simulink model "FixedWing_Dynamic_Model_SIL_simulink"  (R2023a)
settings: Solver=ode4  StartTime=0.0  StopTime=timestop  FixedStep=0.004  RelTol=1e-3
model workspace (MAT data in the model file):
  sample_time = 0.004
values from neighbouring files (symbols this model uses):
  env = struct    [InitEnvironment.m]    (also in resultados_autotuning_H200.mat = )
  F_lat = 1    [autotuning.m]    (also in resultados_autotuning_H200.mat)
  F_lon = 1    [autotuning.m]    (also in resultados_autotuning_H200.mat)
  frecuency = 0.012    [PX4_var_controllers.m]    (also in resultados_autotuning_H200.mat)
  g = 9.81    [PX4_var_controllers.m]    (also in resultados_autotuning_H200.mat)
  LC =     [resultados_autotuning_H200.mat]
  mission = [wp]    [PX4_var_controllers.m]    (also in resultados_autotuning_H200.mat = )
  nav = 0    [autotuning.m]    (also in resultados_autotuning_H200.mat)
  nwap = 9    [PX4_var_controllers.m]    (also in resultados_autotuning_H200.mat)
  pitch_D = p(8)    [Error_Medio_Cuadratico_tot.m]    (also in autotuning.m = gaDat3.xmin(8); resultados_autotuning_H200.mat = 0.0563748318956)
  pitch_ff = p(10)    [Error_Medio_Cuadratico_tot.m]    (also in autotuning.m = gaDat3.xmin(10); resultados_autotuning_H200.mat = 0.191071934851)
  pitch_I = p(7)    [Error_Medio_Cuadratico_tot.m]    (also in autotuning.m = gaDat3.xmin(7); resultados_autotuning_H200.mat = 5.51002123548)
  pitch_P = p(6)    [Error_Medio_Cuadratico_tot.m]    (also in autotuning.m = gaDat3.xmin(6); resultados_autotuning_H200.mat = 0.842081867818)
  poswp = [poswp1;poswp2;poswp3;poswp4;poswp5;poswp6;poswp7;poswp8;poswp9]    [PX4_var_controllers.m]    (also in resultados_autotuning_H200.mat = [0 203.689232032 39.9384744604 259.790159417 479.641844374 3)
  ref_height = 171    [resultados_autotuning_H200.mat]
  ref_lat = 39.4973880749    [resultados_autotuning_H200.mat]
  ref_lon = -0.626812248872    [resultados_autotuning_H200.mat]
  roll_D = p(3)    [Error_Medio_Cuadratico_lat.m]    (also in Error_Medio_Cuadratico_tot.m; autotuning.m = gaDat3.xmin(3); resultados_autotuning_H200.mat = 0.0337053005157)
  roll_ff = p(5)    [Error_Medio_Cuadratico_lat.m]    (also in Error_Medio_Cuadratico_tot.m; autotuning.m = gaDat3.xmin(5); resultados_autotuning_H200.mat = 0.350805641616)
  roll_I = p(2)    [Error_Medio_Cuadratico_lat.m]    (also in Error_Medio_Cuadratico_tot.m; autotuning.m = gaDat3.xmin(2); resultados_autotuning_H200.mat = 5.74910821603)
  roll_P = p(1)    [Error_Medio_Cuadratico_lat.m]    (also in Error_Medio_Cuadratico_tot.m; autotuning.m = gaDat3.xmin(1); resultados_autotuning_H200.mat = 0.613573974385)
  tc_pitch = p(9)    [Error_Medio_Cuadratico_tot.m]    (also in autotuning.m = gaDat3.xmin(9); resultados_autotuning_H200.mat = 0.651709962584)
  tc_roll = p(4)    [Error_Medio_Cuadratico_lat.m]    (also in Error_Medio_Cuadratico_tot.m; autotuning.m = gaDat3.xmin(4); resultados_autotuning_H200.mat = 0.630975334126)
  TEBCL =     [resultados_autotuning_H200.mat]
  TECL =     [resultados_autotuning_H200.mat]
  TECS =     [resultados_autotuning_H200.mat]
  throttle_sp = 0.6    [autotuning.m]    (also in resultados_autotuning_H200.mat)
  uavData = struct    [InitFixedWingParam.m]    (also in resultados_autotuning_H200.mat = )
  V_cruise = [15,15,15,20,25,25,20,15,15]    [PX4_var_controllers.m]    (also in resultados_autotuning_H200.mat = [15 15 15 20 25 25 20 15 15])
  yaw_D = p(8)    [Error_Medio_Cuadratico_lat.m]    (also in Error_Medio_Cuadratico_tot.m = p(13); autotuning.m = gaDat3.xmin(13); resultados_autotuning_H200.mat = 0.366142516918)
  yaw_ff = p(9)    [Error_Medio_Cuadratico_lat.m]    (also in Error_Medio_Cuadratico_tot.m = p(14); autotuning.m = gaDat3.xmin(14); resultados_autotuning_H200.mat = 1.32395168)
  yaw_I = p(7)    [Error_Medio_Cuadratico_lat.m]    (also in Error_Medio_Cuadratico_tot.m = p(12); autotuning.m = gaDat3.xmin(12); resultados_autotuning_H200.mat = 9.97252106698)
  yaw_P = p(6)    [Error_Medio_Cuadratico_lat.m]    (also in Error_Medio_Cuadratico_tot.m = p(11); autotuning.m = gaDat3.xmin(11); resultados_autotuning_H200.mat = 9.79447138521)
undefined symbols (not defined in the file or in its folder): DiscIntNeverNeededParam, Earth, WGS84
libraries: aerolibactuator x5, aerolibasang x4, slpidlib x3, uavalgslib x2, aerolibatmos2 x2, shared6dof x1, aerolibtransform2 x1, simulink_extras x1
(part 1 of 3)
settings Model: Creator=kboychev  LastModifiedBy=user
settings OptimizationCC: ReuseModelBlockBuffer=off  ZeroExternalMemoryAtStartup=off  ZeroInternalMemoryAtStartup=off
settings ModelReferenceCC: EnableRefExpFcnMdlSchedulingChecks=on
settings RTWCC: Toolchain=Microsoft Visual C++ 2017 v15.0 | nmake (64-bit Windows)  TargetLang=C++
settings GRTTargetCC: TargetLangStandard=C++11 (ISO)  CodeInterfacePackaging=C++ class

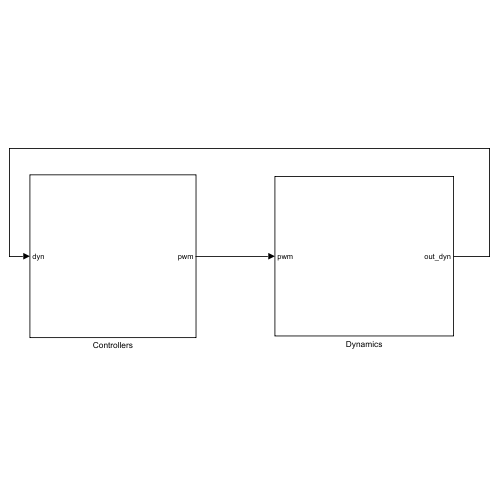
[thumbnail: Simulink's stored preview of the top-level diagram]
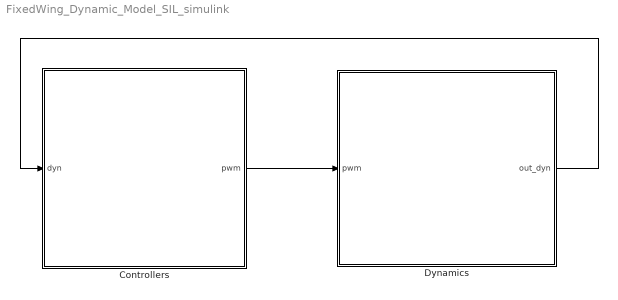
== system FixedWing_Dynamic_Model_SIL_simulink ==
  Controllers : Subsystem
  Dynamics : Subsystem
  wires:
  Dynamics/1(out_dyn) -> Controllers/1(dyn)
  Controllers/1(pwm) -> Dynamics/1(pwm)

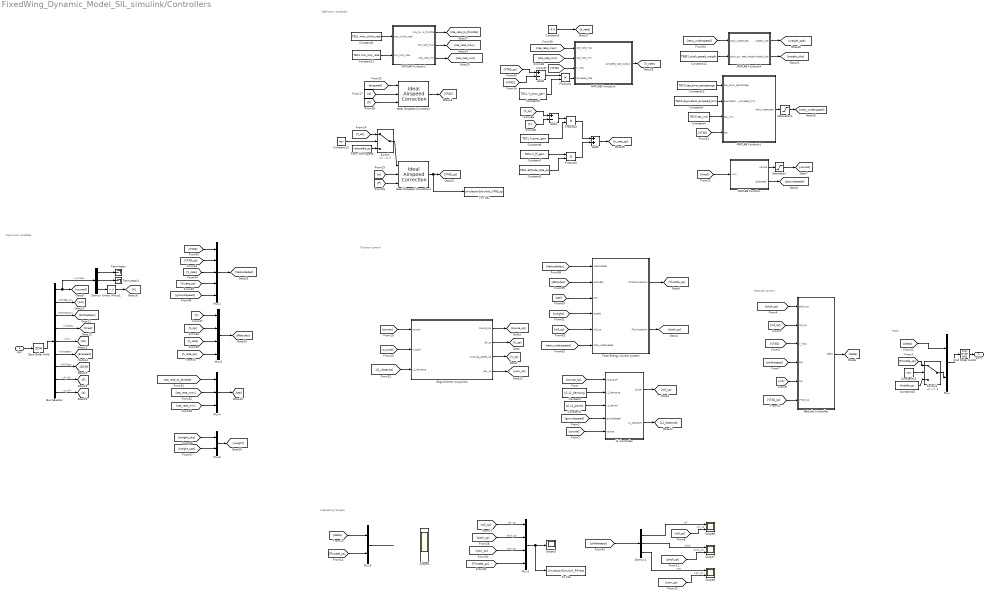
== system FixedWing_Dynamic_Model_SIL_simulink/Controllers ==
  note: Interesting Scopes
  note: Definition Variables
  note: Input and variables
  note: PWM
  note: Attitude control
  note: Position control
  dyn : Inport
  Add3 : Sum  Inputs=+-
  Add4 : Sum  Inputs=+-
  Add5 : Sum
  Attitude Controller : Subsystem
  Bus Selector : BusSelector  OutputSignals=xyzned,omega_b,phithetapsi,Vbned,Vb,airspeed,DCMbe,P_inf,a_inf
  Constant : Constant  Value=LC.L1_damping  SampleTime=frecuency
  Constant1 : Constant  Value=LC.L1_period  SampleTime=frecuency
  Constant10 : Constant  Value=TECS.tas_error_percetange  SampleTime=frecuency
  Constant11 : Constant  Value=TECL.min_sink_rate  SampleTime=frecuency
  Constant12 : Constant  Value=TEBCL.pitch_speed_weight  SampleTime=frecuency
  Constant13 : Constant  Value=nav  SampleTime=frecuency
  Constant15 : Constant  Value=nav  SampleTime=frecuency
  Constant16 : Constant  Value=throttle_sp  SampleTime=frecuency
  Constant2 : Constant  Value=TECL.altitude_rate_sp  SampleTime=frecuency
  Constant3 : Constant  Value=-0.5  SampleTime=frecuency
  Constant4 : Constant  Value=TECS.tas_min  SampleTime=frecuency
  Constant5 : Constant  Value=TECL.V_error_gain  SampleTime=frecuency
  Constant6 : Constant  Value=TECL.h_error_gain  SampleTime=frecuency
  Constant7 : Constant  Value=TECL.h_ff_gain  SampleTime=frecuency
  Constant8 : Constant  Value=TECL.max_climb_rate  SampleTime=frecuency
  Constant9 : Constant  Value=TECS.equivalent_airspeed_trim  SampleTime=frecuency
  Demux : Demux  Outputs=3
  Demux1 : Demux  Outputs=3
  First Order Hold1 : FirstOrderHold  ErrorTolerance=inf  AllowContinuousInput=on
  From Workspace : FromWorkspace  VariableName=velocidad_sp  SampleTime=frecuency
  Ideal Airspeed Correction : aerolibasang/Ideal Airspeed Correction  units=Metric (MKS)  vel_in=EAS  vel_out_tas=EAS  vel_out_eas=TAS  vel_out_cas=TAS  method=Table Lookup  SubOnly=off  action=None
  Ideal Airspeed Correction1 : aerolibasang/Ideal Airspeed Correction  units=Metric (MKS)  vel_in=EAS  vel_out_tas=EAS  vel_out_eas=TAS  vel_out_cas=TAS  method=Table Lookup  SubOnly=off  action=None
  L1 Controller : Subsystem
  MATLAB Function : MATLAB Function  TreatAsAtomicUnit=on  SystemSampleTime=frecuency
  MATLAB Function1 : MATLAB Function  TreatAsAtomicUnit=on  SystemSampleTime=frecuency
  MATLAB Function2 : MATLAB Function  TreatAsAtomicUnit=on  SystemSampleTime=frecuency
  MATLAB Function3 : MATLAB Function  TreatAsAtomicUnit=on  SystemSampleTime=frecuency
  MATLAB Function4 : MATLAB Function  TreatAsAtomicUnit=on  SystemSampleTime=frecuency
  Mux : Mux  Inputs=2
  Mux1 : Mux
  Mux2 : Mux  Inputs=5
  Mux3 : Mux
  Mux4 : Mux  Inputs=3
  Mux5 : Mux  Inputs=2
  Mux6 : Mux  Inputs=2
  Product2 : Product
  Product3 : Product
  Product4 : Product
  Saturation : Saturate  UpperLimit=pi  LowerLimit=-pi
  Saturation1 : Saturate  UpperLimit=1  LowerLimit=0
  Scope3 : Scope
  Scope4 : Scope  NumInputPorts=4
  Scope6 : Scope  NumInputPorts=2
  Scope7 : Scope  NumInputPorts=2
  Scope8 : Scope  NumInputPorts=2
  Seguimiento waypoints : Subsystem
  Switch : Switch  Criteria=u2 ~= 0  SaturateOnIntegerOverflow=off  InputSameDT=off
  Switch1 : Switch  Criteria=u2 ~= 0  SaturateOnIntegerOverflow=off  InputSameDT=off
  Terminator : Terminator
  Terminator1 : Terminator
  To File : ToFile  Filename=simulacionSimulink_RPYest  SaveFormat=Timeseries
  To File1 : ToFile  Filename=simulacionSimulink_VTAS_sp  SaveFormat=Timeseries
  Total Energy control system : Subsystem
  Unary Minus1 : UnaryMinus
  Zero-Order Hold : ZeroOrderHold  SampleTime=frecuency
  pwm : Outport
  wires:
  Seguimiento waypoints/2(alt_sp) -> [h_sp]
  Seguimiento waypoints/3(cruising_speed_sp) -> [V_sp]
  Seguimiento waypoints/1(Course_sp) -> [course_sp]
  [course] -> L1 Controller/5(course)
  Total Energy control system/1(Throttle setpoint) -> [Throttle_sp]
  Total Energy control system/2(Pitch setpoint) -> [pitch_sp]
  [pitch_sp] -> Attitude Controller/1(pitch_sp)
  [roll_sp] -> Attitude Controller/2(roll_sp)
  [VTAS] -> Attitude Controller/3(V_TAS)
  [phithetapsi] -> Attitude Controller/4("RPY ")
  [wb] -> Attitude Controller/5(wb)
  [VTAS_sp] -> Attitude Controller/6(VTAS_sp)
  Attitude Controller/1(delta) -> [delta]
  [course] -> Seguimiento waypoints/1(course)
  [xyzned] -> Seguimiento waypoints/2(xyzgnd)
  MATLAB Function/1(course) -> Saturation/1
  Bus Selector/1 -> Demux/1, [xyzned]  "<xyzned>"
  Bus Selector/2 -> [wb]  "<omega_b>"
  Bus Selector/3 -> [phithetapsi]  "<phithetapsi>"
  Bus Selector/4 -> [Vned]  "<Vbned>"
  Bus Selector/5 -> [Vb]  "<Vb>"
  Bus Selector/6 -> [airspeed]  "<airspeed>"
  Bus Selector/7 -> [DCM]  "<DCMbe>"
  Bus Selector/8 -> [P]  "<P_inf>"
  Bus Selector/9 -> [a]  "<a_inf>"
  [a] -> Ideal Airspeed Correction/2
  [P] -> Ideal Airspeed Correction/3
  [airspeed] -> Ideal Airspeed Correction/1
  [P] -> Ideal Airspeed Correction1/3
  [a] -> Ideal Airspeed Correction1/2
  Ideal Airspeed Correction1/1 -> To File1/1, [VTAS_sp]
  Demux/1 -> Terminator/1
  Demux/2 -> Terminator1/1
  Demux/3 -> Unary Minus1/1
  Unary Minus1/1 -> [h]
  L1 Controller/2(L1_distance) -> [L1_distance]
  L1 Controller/1(roll SP) -> [roll_sp]
  [groundspeed] -> L1 Controller/4(groundSpeed)
  MATLAB Function/2(gndspeed) -> [groundspeed]
  Seguimiento waypoints/4(yaw_sp) -> [yaw_sp]
  [roll_sp] -> Mux1/1  "roll_sp"
  [pitch_sp] -> Mux1/2  "pitch_sp"
  [yaw_sp] -> Mux1/3  "yaw_sp"
  [Throttle_sp] -> Mux1/4
  Ideal Airspeed Correction/1 -> [VTAS]
  Mux1/1 -> Scope3/1, To File/1
  Saturation/1 -> [course]
  [Vned] -> MATLAB Function/1(vxyz)
  Demux1/2 -> Scope7/1  "pitch"
  Demux1/3 -> Scope8/1  "yaw"
  dyn/1 -> Zero-Order Hold/1
  Mux/1 -> First Order Hold1/1
  Zero-Order Hold/1 -> Bus Selector/1
  Constant/1 -> L1 Controller/2(L1_damping)
  Constant1/1 -> L1 Controller/3(L1_period)
  Demux1/1 -> Scope6/1  "roll"
  First Order Hold1/1 -> pwm/1
  [delta] -> Mux/1
  [course_sp] -> L1 Controller/1(course SP)
  [L1_distance] -> Seguimiento waypoints/3(L1_distance)
  Saturation1/1 -> [ratio_underspeed]
  Constant9/1 -> MATLAB Function1/2(equivalent_airspeed_trim)
  Constant8/1 -> MATLAB Function2/1(max_climb_rate)
  Constant4/1 -> MATLAB Function1/3(tas_min)
  Constant10/1 -> MATLAB Function1/1(tas_error_percentage)
  MATLAB Function1/1(ratio_undersped) -> Saturation1/1
  Constant11/1 -> MATLAB Function2/2(min_sink_rate)
  [VTAS] -> MATLAB Function1/4(tas)
  MATLAB Function2/2(ste_rate_max) -> [ste_rate_max]
  MATLAB Function2/3(ste_rate_min) -> [ste_rate_min]
  MATLAB Function2/1(ste_rate_to_throttle) -> [ste_rate_to_throttle]
  [VTAS] -> MATLAB Function3/3(V_TAS)
  [ste_rate_max] -> MATLAB Function3/1(ste_rate_max)
  [h] -> Add4/2
  [ste_rate_min] -> MATLAB Function3/2(ste_rate_min)
  Constant5/1 -> Product2/2
  Constant6/1 -> Product3/2
  Product4/1 -> Add5/2
  [h_sp] -> Add4/1
  Add3/1 -> Product2/1
  Product2/1 -> MATLAB Function3/4(airspeed_rate)
  [VTAS] -> Add3/2
  Product3/1 -> Add5/1
  Constant7/1 -> Product4/1
  [VTAS_sp] -> Add3/1
  Constant2/1 -> Product4/2
  Add4/1 -> Product3/1
  MATLAB Function3/1(airspeed_rate_output) -> [V_rate]
  [ratio_underspeed] -> MATLAB Function4/1(ratio_undersped)
  Constant12/1 -> MATLAB Function4/2(pitch_speed_weight)
  MATLAB Function4/1(weight_spe) -> [weight_spe]
  MATLAB Function4/2(weight_ske) -> [weight_ske]
  [phithetapsi] -> Demux1/1
  Mux2/1 -> [Velocidades]
  [VTAS] -> Mux2/1
  [VTAS_sp] -> Mux2/2
  [V_rate] -> Mux2/3
  [V_rate_sp] -> Mux2/4
  [groundspeed] -> Mux2/5
  Mux3/1 -> [Altitudes]
  [h] -> Mux3/1
  [h_sp] -> Mux3/2
  [h_rate] -> Mux3/3
  [h_rate_sp] -> Mux3/4
  Mux4/1 -> [ste]
  [ste_rate_to_throttle] -> Mux4/1
  [ste_rate_max] -> Mux4/2
  [ste_rate_min] -> Mux4/3
  Mux6/1 -> [weight]
  [weight_spe] -> Mux6/2
  [weight_ske] -> Mux6/1
  [Velocidades] -> Total Energy control system/1(Velocidades)
  [Altitudes] -> Total Energy control system/2(Altitudes)
  [ste] -> Total Energy control system/3(ste)
  [weight] -> Total Energy control system/4(weight)
  [roll_sp] -> Total Energy control system/5(roll_sp)
  [ratio_underspeed] -> Total Energy control system/6(ratio_underspeed)
  Add5/1 -> [h_rate_sp]
  Constant3/1 -> [h_rate]
  [roll_sp] -> Scope6/2  "roll_sp"
  [pitch_sp] -> Scope7/2  "pitch_sp"
  [yaw_sp] -> Scope8/2  "yaw_sp"
  Mux5/1 -> ?
  [delta] -> Mux5/1
  [Throttle_sp] -> Mux5/2
  ? -> Scope4/3  "dR"
  ? -> Scope4/1  "dE"
  ? -> Scope4/2  "dA"
  ? -> Scope4/4  "dT"
  [V_sp] -> Switch/1
  Switch/1 -> Ideal Airspeed Correction1/1
  Constant13/1 -> Switch/2
  From Workspace/1 -> Switch/3
  Constant16/1 -> Switch1/3
  Constant15/1 -> Switch1/2
  [Throttle_sp] -> Switch1/1
  Switch1/1 -> Mux/2

== system FixedWing_Dynamic_Model_SIL_simulink/Dynamics ==
  note: Pixhawk SIL Connector for Simulink
      | Fixed-Wing Dynamics
  pwm : Inport
  Bus Selector : BusSelector  OutputSignals=mulh,phithetapsi,Vbned,xyzned,Vb,omega_b,g,B
  Demux : Demux  Outputs=3
  Display{,1..5,10..11,13} (9 alike) : Display
  H200 Fixed-wing UAV Dynamics : Subsystem
  Radians to Degrees2 : simulink_extras/Transformations/Radians to Degrees
  Scope2 : Scope
  Unary Minus : UnaryMinus
  XY Graph : Record  FileSettingsInternal="{\"entries\":[{\"content\":{\"excelSettings\":{\"content\":{},\"type\":\"Streamout.ExcelSettings\"}},\"type\":\"Streamout.FileSettingStorage\",\"uuid\":\"\"}],\"packageUris\":[\"http:\\/\\/schema.mathworks.com\\/mf0\\/streamout_blocks\\/R2020a\"],\"version\":\"1.0\"}"  Layout=[1 1]  SignalsInternal="{\"entries\":[{\"content\":{\"signals\":[{\"content\":{\"blockPath\":[],\"dimensions\":[1],\"domain\":\"\",\"lineColor\":\"#a2142f\",\"plots\":[1],\"port\":1,\"signalID\":86,\"signalName\":\"Demux:2\"},\"type\":\"RecordBlkView.Signal\",\"uuid\":\"\"},{\"content\":{\"blockPath\":[],\"dimensions\":[1],\"domain\":\"\",\"lineColor\":\"#139fff\",\"plots\":[1],\"port\":2,\"signalID\":89,\"signalName\":\"Demux:1\"},\"type\":\"RecordBlkView.Signal\",\"uuid\":\"\"}]},\"type\":\"RecordBlkView.InputSignals\",\"uuid\":\"\"}],\"packageUris\":[\"http:\\/\\/schema.mathworks.com\\/mf0\\/streamout_blocks\\/R2020a\"],\"version\":\"1.0\"}"  VisualizationBindings="{\"xyplotplugin\":{\"info\":[{\"series\":[{\"bindingParametersList\":[{\"parameter\":\"X-Axis\",\"signalID\":86,\"signalName\":\"Demux:2\"},{\"parameter\":\"Y-Axis\",\"signalID\":89,\"signalName\":\"Demux:1\"}],\"seriesID\":12918}],\"subplotID\":1}]}}"  CompatibilityTag=XY
  XY Graph1 : Record  FileSettingsInternal="{\"entries\":[{\"content\":{\"excelSettings\":{\"content\":{},\"type\":\"Streamout.ExcelSettings\"}},\"type\":\"Streamout.FileSettingStorage\",\"uuid\":\"\"}],\"packageUris\":[\"http:\\/\\/schema.mathworks.com\\/mf0\\/streamout_blocks\\/R2020a\"],\"version\":\"1.0\"}"  Layout=[1 1]  SignalsInternal="{\"entries\":[{\"content\":{\"signals\":[{\"content\":{\"blockPath\":[],\"dimensions\":[1],\"domain\":\"\",\"lineColor\":\"#a2142f\",\"plots\":[1],\"port\":1,\"signalID\":78,\"signalName\":\"Demux:1\"},\"type\":\"RecordBlkView.Signal\",\"uuid\":\"\"},{\"content\":{\"blockPath\":[],\"dimensions\":[1],\"domain\":\"\",\"lineColor\":\"#139fff\",\"plots\":[1],\"port\":2,\"signalID\":81,\"signalName\":\"Unary Minus\"},\"type\":\"RecordBlkView.Signal\",\"uuid\":\"\"}]},\"type\":\"RecordBlkView.InputSignals\",\"uuid\":\"\"}],\"packageUris\":[\"http:\\/\\/schema.mathworks.com\\/mf0\\/streamout_blocks\\/R2020a\"],\"version\":\"1.0\"}"  VisualizationBindings="{\"xyplotplugin\":{\"info\":[{\"series\":[{\"bindingParametersList\":[{\"parameter\":\"X-Axis\",\"signalID\":78,\"signalName\":\"Demux:1\"},{\"parameter\":\"Y-Axis\",\"signalID\":81,\"signalName\":\"Unary Minus\"}],\"seriesID\":30530}],\"subplotID\":1}]}}"  CompatibilityTag=XY
  save to file : Subsystem
  out_dyn : Outport
  wires:
  Bus Selector/4 -> Demux/1, Display10/1  "<xyzned>"
  Radians to Degrees2/1 -> Display1/1, Scope2/1
  Bus Selector/1 -> Display/1  "<mulh>"
  Bus Selector/5 -> Display3/1  "<Vb>"
  Bus Selector/7 -> Display13/1  "<g>"
  Bus Selector/8 -> Display11/1  "<B>"
  Bus Selector/3 -> Display2/1  "<Vbned>"
  Bus Selector/6 -> Display4/1  "<omega_b>"
  Bus Selector/2 -> Radians to Degrees2/1  "<phithetapsi>"
  H200 Fixed-wing UAV Dynamics/1(out) -> out_dyn/1, save to file/2(out), Bus Selector/1
  Demux/1 -> XY Graph/2, XY Graph1/1
  Demux/3 -> Unary Minus/1
  Unary Minus/1 -> XY Graph1/2
  Demux/2 -> XY Graph/1
  pwm/1 -> H200 Fixed-wing UAV Dynamics/1(pwm), Display5/1, save to file/1(pwm)

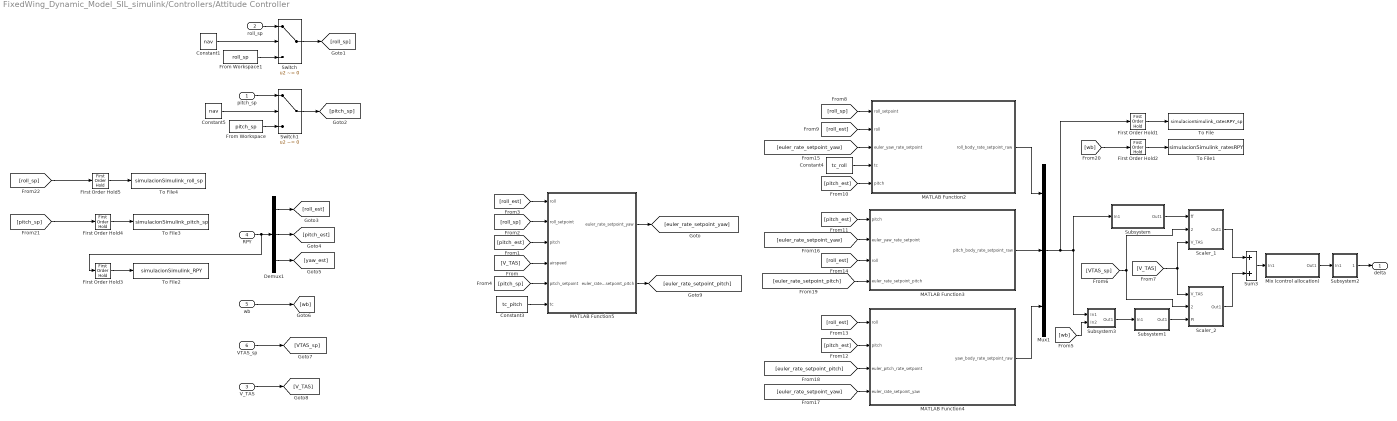
== system FixedWing_Dynamic_Model_SIL_simulink/Controllers/Attitude Controller ==
  pitch_sp : Inport  SampleTime=frecuency
  roll_sp : Inport  Port=2  SampleTime=frecuency
  V_TAS : Inport  Port=3  SampleTime=frecuency
  "RPY " : Inport  Port=4  SampleTime=frecuency
  wb : Inport  Port=5  SampleTime=frecuency
  VTAS_sp : Inport  Port=6  SampleTime=frecuency
  Constant1 : Constant  Value=nav  SampleTime=frecuency
  Constant3 : Constant  Value=tc_pitch  SampleTime=frecuency
  Constant4 : Constant  Value=tc_roll  SampleTime=frecuency
  Constant5 : Constant  Value=nav  SampleTime=frecuency
  Demux1 : Demux  Outputs=3
  First Order Hold{1..5} (5 alike) : FirstOrderHold  ErrorTolerance=inf  AllowContinuousInput=on
  From Workspace : FromWorkspace  VariableName=pitch_sp  SampleTime=frecuency
  From Workspace1 : FromWorkspace  VariableName=roll_sp  SampleTime=frecuency
  MATLAB Function2 : MATLAB Function  TreatAsAtomicUnit=on  SystemSampleTime=frecuency
  MATLAB Function3 : MATLAB Function  TreatAsAtomicUnit=on  SystemSampleTime=frecuency
  MATLAB Function4 : MATLAB Function  TreatAsAtomicUnit=on  SystemSampleTime=frecuency
  MATLAB Function5 : MATLAB Function  TreatAsAtomicUnit=on  SystemSampleTime=frecuency
  Mix (control allocation) : Subsystem
  Mux1 : Mux  Inputs=3
  Scaler_1 : Subsystem
  Scaler_2 : Subsystem
  Subsystem : Subsystem
  Subsystem1 : Subsystem
  Subsystem2 : Subsystem
  Subsystem3 : Subsystem
  Sum3 : Sum
  Switch : Switch  Criteria=u2 ~= 0  SaturateOnIntegerOverflow=off  InputSameDT=off
  Switch1 : Switch  Criteria=u2 ~= 0  SaturateOnIntegerOverflow=off  InputSameDT=off
  To File : ToFile  Filename=simulacionSimulink_ratesRPY_sp  SaveFormat=Timeseries
  To File1 : ToFile  Filename=simulacionSimulink_ratesRPY  SaveFormat=Timeseries
  To File2 : ToFile  Filename=simulacionSimulink_RPY  SaveFormat=Timeseries
  To File3 : ToFile  Filename=simulacionSimulink_pitch_sp  SaveFormat=Timeseries
  To File4 : ToFile  Filename=simulacionSimulink_roll_sp  SaveFormat=Timeseries
  delta : Outport  SampleTime=frecuency
  wires:
  Scaler_1/1(Out1) -> Sum3/1
  Subsystem3/1(Out1) -> Subsystem1/1(In1)
  Subsystem/1(Out1) -> Scaler_1/1(ff)
  Mix (control allocation)/1(Out1) -> Subsystem2/1(In1)
  Sum3/1 -> Mix (control allocation)/1(In1)
  Subsystem2/1(Out1) -> delta/1
  Scaler_2/1(Out1) -> Sum3/2
  Subsystem1/1(Out1) -> Scaler_2/3(PI)
  "RPY "/1 -> First Order Hold3/1, Demux1/1
  Constant3/1 -> MATLAB Function5/6(tc)
  Constant4/1 -> MATLAB Function2/4(tc)
  [V_TAS] -> MATLAB Function5/4(airspeed)
  MATLAB Function2/1(roll_body_rate_setpoint_raw) -> Mux1/1
  MATLAB Function3/1(pitch_body_rate_setpoint_raw) -> Mux1/2
  MATLAB Function4/1(yaw_body_rate_setpoint_raw) -> Mux1/3
  Mux1/1 -> First Order Hold1/1, Subsystem3/1(In1), Subsystem/1(In1)
  First Order Hold1/1 -> To File/1
  Demux1/1 -> [roll_est]
  Demux1/2 -> [pitch_est]
  Demux1/3 -> [yaw_est]
  wb/1 -> [wb]
  VTAS_sp/1 -> [VTAS_sp]
  V_TAS/1 -> [V_TAS]
  [roll_est] -> MATLAB Function5/1(roll)
  [roll_sp] -> MATLAB Function5/2(roll_setpoint)
  [pitch_est] -> MATLAB Function5/3(pitch)
  [pitch_sp] -> MATLAB Function5/5(pitch_setpoint)
  [wb] -> Subsystem3/2(In2)
  [VTAS_sp] -> Scaler_2/2(VTAS_sp), Scaler_1/2(VTAS_sp)
  [V_TAS] -> Scaler_2/1(V_TAS), Scaler_1/3(V_TAS)
  MATLAB Function5/2(euler_rate_setpoint_pitch) -> [euler_rate_setpoint_pitch]
  MATLAB Function5/1(euler_rate_setpoint_yaw) -> [euler_rate_setpoint_yaw]
  [roll_sp] -> MATLAB Function2/1(roll_setpoint)
  [roll_est] -> MATLAB Function2/2(roll)
  [pitch_est] -> MATLAB Function2/5(pitch)
  [pitch_est] -> MATLAB Function3/1(pitch)
  [pitch_est] -> MATLAB Function4/2(pitch)
  [roll_est] -> MATLAB Function4/1(roll)
  [roll_est] -> MATLAB Function3/3(roll)
  [euler_rate_setpoint_yaw] -> MATLAB Function2/3(euler_yaw_rate_setpoint)
  [euler_rate_setpoint_yaw] -> MATLAB Function3/2(euler_yaw_rate_setpoint)
  [euler_rate_setpoint_yaw] -> MATLAB Function4/4(euler_rate_setpoint_yaw)
  [euler_rate_setpoint_pitch] -> MATLAB Function3/4(euler_rate_setpoint_pitch)
  [euler_rate_setpoint_pitch] -> MATLAB Function4/3(euler_pitch_rate_setpoint)
  First Order Hold2/1 -> To File1/1
  [wb] -> First Order Hold2/1
  First Order Hold3/1 -> To File2/1
  First Order Hold4/1 -> To File3/1
  [roll_sp] -> First Order Hold5/1
  First Order Hold5/1 -> To File4/1
  [pitch_sp] -> First Order Hold4/1
  roll_sp/1 -> Switch/1
  Switch/1 -> [roll_sp]
  From Workspace1/1 -> Switch/3
  Constant1/1 -> Switch/2
  Switch1/1 -> [pitch_sp]
  pitch_sp/1 -> Switch1/1
  Constant5/1 -> Switch1/2
  From Workspace/1 -> Switch1/3

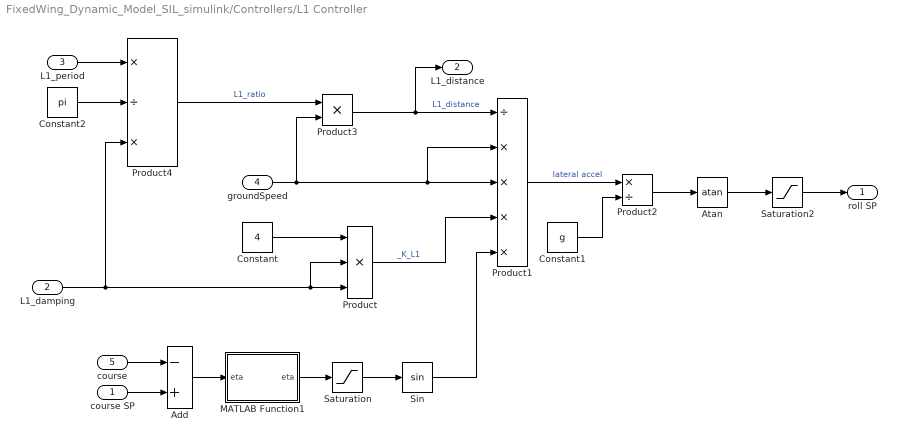
== system FixedWing_Dynamic_Model_SIL_simulink/Controllers/L1 Controller ==
  course SP : Inport  SampleTime=frecuency
  L1_damping : Inport  Port=2  SampleTime=frecuency
  L1_period : Inport  Port=3  SampleTime=frecuency
  groundSpeed : Inport  Port=4  SampleTime=frecuency
  course : Inport  Port=5  SampleTime=frecuency
  Add : Sum  Inputs=-+
  Atan : Trigonometry  Operator=atan
  Constant : Constant  Value=4  SampleTime=frecuency
  Constant1 : Constant  Value=g  SampleTime=frecuency
  Constant2 : Constant  Value=pi  SampleTime=frecuency
  MATLAB Function1 : MATLAB Function  TreatAsAtomicUnit=on  SystemSampleTime=frecuency
  Product : Product  Inputs=3
  Product1 : Product  Inputs=/****
  Product2 : Product  Inputs=*/
  Product3 : Product
  Product4 : Product  Inputs=*/*
  Saturation : Saturate  UpperLimit=pi/2  LowerLimit=-pi/2
  Saturation2 : Saturate  UpperLimit=LC.roll_max  LowerLimit=LC.roll_min
  Sin : Trigonometry
  roll SP : Outport  SampleTime=frecuency
  L1_distance : Outport  Port=2  SampleTime=frecuency
  wires:
  Constant/1 -> Product/1
  L1_damping/1 -> Product4/3, Product/3, Product/2
  groundSpeed/1 -> Product3/2, Product1/2, Product1/3
  Product/1 -> Product1/4  "_K_L1"
  Product1/1 -> Product2/1  "lateral accel"
  Product2/1 -> Atan/1
  Product4/1 -> Product3/1  "L1_ratio"
  L1_period/1 -> Product4/1
  Constant2/1 -> Product4/2
  Constant1/1 -> Product2/2
  Atan/1 -> Saturation2/1
  Sin/1 -> Product1/5
  Product3/1 -> L1_distance/1, Product1/1  "L1_distance"
  Saturation2/1 -> roll SP/1
  Add/1 -> MATLAB Function1/1("eta ")
  MATLAB Function1/1(eta) -> Saturation/1
  Saturation/1 -> Sin/1
  course/1 -> Add/1
  course SP/1 -> Add/2

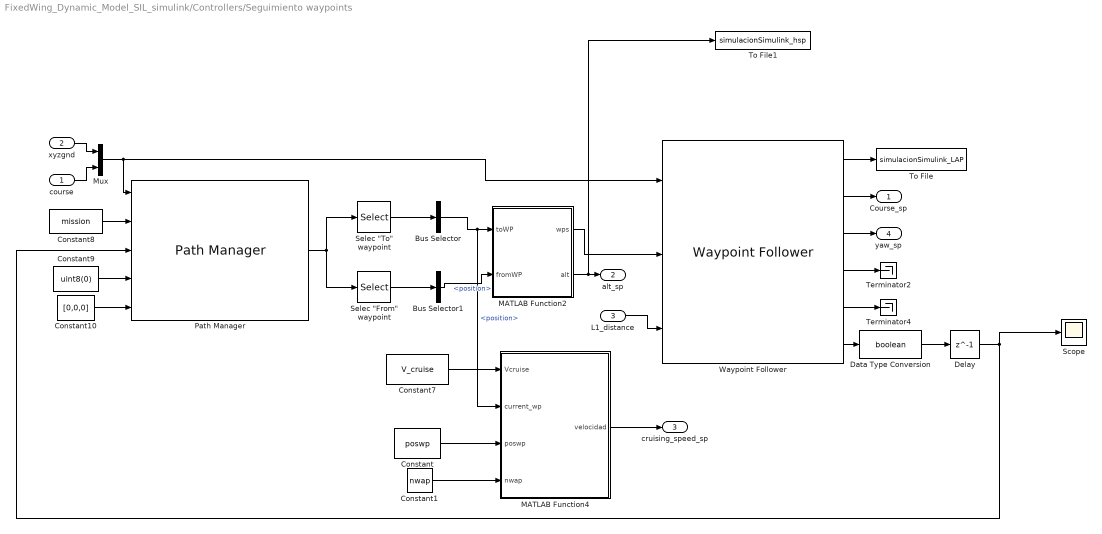
== system FixedWing_Dynamic_Model_SIL_simulink/Controllers/Seguimiento waypoints ==
  course : Inport  SampleTime=frecuency
  xyzgnd : Inport  Port=2  SampleTime=frecuency
  L1_distance : Inport  Port=3  SampleTime=frecuency
  Bus Selector : BusSelector  OutputSignals=position
  Bus Selector1 : BusSelector  OutputSignals=position
  Constant : Constant  Value=poswp  SampleTime=frecuency
  Constant1 : Constant  Value=nwap  SampleTime=frecuency
  Constant10 : Constant  Value=[0,0,0]  SampleTime=frecuency
  Constant7 : Constant  Value=V_cruise  SampleTime=frecuency
  Constant8 : Constant  Value=mission  OutDataTypeStr=Bus: UAVPathManagerBus  SampleTime=frecuency
  Constant9 : Constant  Value=uint8(0)  SampleTime=frecuency
  Data Type Conversion : DataTypeConversion  OutDataTypeStr=boolean  SaturateOnIntegerOverflow=off  RndMeth=Floor
  Delay : Delay  DelayLength=1  SampleTime=frecuency
  MATLAB Function2 : MATLAB Function  TreatAsAtomicUnit=on  SystemSampleTime=frecuency
  MATLAB Function4 : MATLAB Function  TreatAsAtomicUnit=on  SystemSampleTime=frecuency
  Mux : Mux  Inputs=2
  Path Manager : uavalgslib/Path Manager  UAVType=fixed-wing  LoiterRadius=transitionRadius  dataType=double  inputBusName='UAVPathManagerBus'  SimulateUsing=Interpreted execution
  Scope : Scope
  "Selec \"From\" waypoint" : Selector  InputPortWidth=2  IndexOptions=Index vector (dialog)  Indices=2  OutputSizes=1
  "Selec \"To\" waypoint" : Selector  InputPortWidth=2  IndexOptions=Index vector (dialog)  Indices=1  OutputSizes=1
  Terminator2 : Terminator
  Terminator4 : Terminator
  To File : ToFile  Filename=simulacionSimulink_LAP  SaveFormat=Timeseries
  To File1 : ToFile  Filename=simulacionSimulink_hsp  SaveFormat=Timeseries
  Waypoint Follower : uavalgslib/Waypoint Follower  UAVType=fixed-wing  StartFrom=first  TransitionRadiusSource=internal  TransitionRadius=transitionRadius  MinLookaheadDistance=20  YawInput=off  ShowCrossTrackErrorOutput=on  ShowStatusOutput=on  SimulateUsing=Interpreted execution
  Course_sp : Outport  SampleTime=frecuency
  alt_sp : Outport  Port=2  SampleTime=frecuency
  cruising_speed_sp : Outport  Port=3  SampleTime=frecuency
  yaw_sp : Outport  Port=4  SampleTime=frecuency
  wires:
  Waypoint Follower/2 -> Course_sp/1
  Waypoint Follower/4 -> Terminator2/1
  course/1 -> Mux/2
  MATLAB Function2/2(alt) -> To File1/1, alt_sp/1
  Path Manager/1 -> "Selec \"To\" waypoint"/1, "Selec \"From\" waypoint"/1
  "Selec \"To\" waypoint"/1 -> Bus Selector/1
  "Selec \"From\" waypoint"/1 -> Bus Selector1/1
  Bus Selector/1 -> MATLAB Function4/2(current_wp), MATLAB Function2/1(toWP)  "<position>"
  Bus Selector1/1 -> MATLAB Function2/2(fromWP)  "<position>"
  Waypoint Follower/1 -> To File/1
  Delay/1 -> Scope/1, Path Manager/3
  Data Type Conversion/1 -> Delay/1
  L1_distance/1 -> Waypoint Follower/3
  Waypoint Follower/6 -> Data Type Conversion/1
  Waypoint Follower/5 -> Terminator4/1
  Waypoint Follower/3 -> yaw_sp/1
  Constant8/1 -> Path Manager/2
  Constant9/1 -> Path Manager/4
  Constant10/1 -> Path Manager/5
  Constant7/1 -> MATLAB Function4/1(Vcruise)
  xyzgnd/1 -> Mux/1
  Mux/1 -> Waypoint Follower/1, Path Manager/1
  MATLAB Function2/1(wps) -> Waypoint Follower/2
  MATLAB Function4/1(velocidad) -> cruising_speed_sp/1
  Constant1/1 -> MATLAB Function4/4(nwap)
  Constant/1 -> MATLAB Function4/3(poswp)

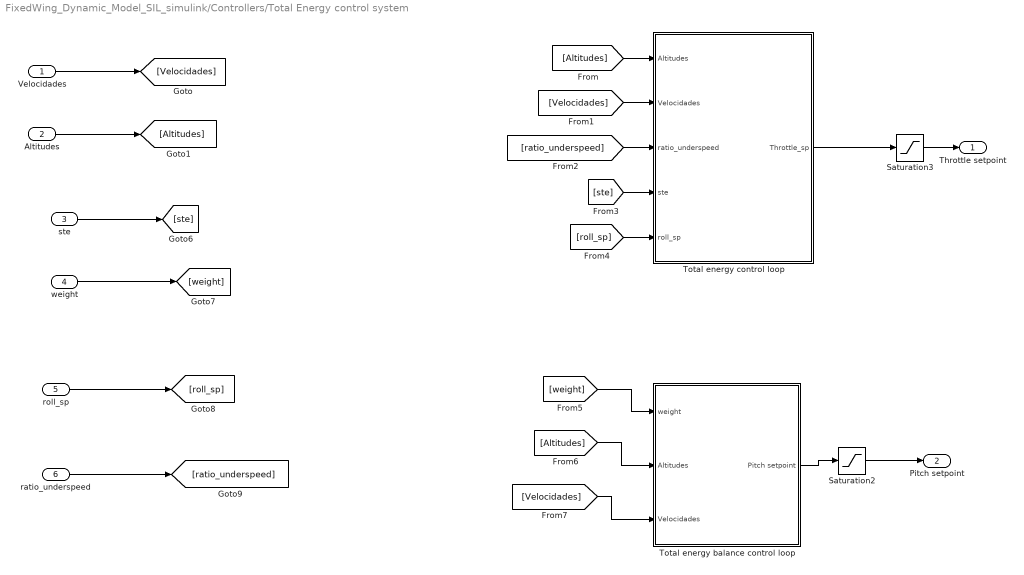
== system FixedWing_Dynamic_Model_SIL_simulink/Controllers/Total Energy control system ==
  Velocidades : Inport  SampleTime=frecuency
  Altitudes : Inport  Port=2  SampleTime=frecuency
  ste : Inport  Port=3  SampleTime=frecuency
  weight : Inport  Port=4  SampleTime=frecuency
  roll_sp : Inport  Port=5  SampleTime=frecuency
  ratio_underspeed : Inport  Port=6  SampleTime=frecuency
  Saturation2 : Saturate  UpperLimit=TEBCL.pitch_max  LowerLimit=TEBCL.pitch_min
  Saturation3 : Saturate  UpperLimit=TECL.T_max  LowerLimit=TECL.T_min
  Total energy balance control loop : Subsystem
  Total energy control loop : Subsystem
  Throttle setpoint : Outport  SampleTime=frecuency
  Pitch setpoint : Outport  Port=2  SampleTime=frecuency
  wires:
  Total energy balance control loop/1(Pitch setpoint) -> Saturation2/1
  Total energy control loop/1(Throttle_sp) -> Saturation3/1
  Saturation3/1 -> Throttle setpoint/1
  Saturation2/1 -> Pitch setpoint/1
  Velocidades/1 -> [Velocidades]
  Altitudes/1 -> [Altitudes]
  ste/1 -> [ste]
  weight/1 -> [weight]
  roll_sp/1 -> [roll_sp]
  ratio_underspeed/1 -> [ratio_underspeed]
  [Altitudes] -> Total energy control loop/1(Altitudes)
  [Velocidades] -> Total energy control loop/2(Velocidades)
  [ratio_underspeed] -> Total energy control loop/3(ratio_underspeed)
  [ste] -> Total energy control loop/4(ste)
  [roll_sp] -> Total energy control loop/5(roll_sp)
  [weight] -> Total energy balance control loop/1(weight)
  [Altitudes] -> Total energy balance control loop/2(Altitudes)
  [Velocidades] -> Total energy balance control loop/3(Velocidades)

== system FixedWing_Dynamic_Model_SIL_simulink/Dynamics/H200 Fixed-wing UAV Dynamics ==
  note: Note:
      | DCM_be converts a vector written in earth frame to body frame
      | Abe is acceleration of body written in body frame, but measured relative to earth.
      | To get acceleration of body written in earth frame (NED fixed on takeoff location), we need to convert the frame.
      | IMU block's angular velocity and acceleration inputs are written in earth frame (NED)
  pwm : Inport
  "6DOF Rigid body dynamics " : shared6dof/6DOF (Euler Angles)  units=Metric (MKS)  mtype=Fixed  rep=Quaternion  xme_0=init.posNED  Vm_0=init.vb  eul_0=init.euler  pm_0=init.angRates  mass_0=uavData.geometry.m  mass_e=0.5  mass_f=2.0  inertia=diag([uavData.inertia.Ixx, uavData.inertia.Iyy, uavData.inertia.Izz])  inertia_e=eye(3)  inertia_f=2*eye(3)  k_quat=1  vre_flag=on  abi_flag=on  aMode=aMode  xme_statename=''  Vm_statename=''  eul_statename=''  quat_statename=''  pm_statename=''  mass_statename=''
  Bus Creator : BusCreator  Inputs=16
  Constant : Constant  Value=- ref_height
  Constant1 : Constant  Value=[0 0 env.ISA_g]'
  Constant2 : Constant  Value=[21.5 1.16 43.1]
  Constant3 : Constant  Value=env.windVector
  Flat Earth to LLA : aerolibtransform2/Flat Earth to LLA  units=Metric (MKS)  ptype=Earth (WGS84)  F=1/298.257223563  R=6378137  refPosPort=off  LL0=[ref_lat, ref_lon]  psi=0
  Force and Moment Calculation : Subsystem
  ISA Atmosphere Model : aerolibatmos2/ISA Atmosphere Model  custom=on  g=env.ISA_g  gamma=env.ISA_ratioHeats  R=env.ISA_R  L=env.ISA_lapse  h_trop=env.ISA_troposphereHeight  h_strat=env.ISA_tropopauseHeight  rho0=env.ISA_rho0  P0=env.ISA_P0  T0=env.ISA_T0  h0=env.ISA_hmin
  Mux : Mux  Inputs=2
  Selector : Selector  IndexMode=Zero-based  InputPortWidth=3  IndexOptions=Index vector (dialog)  Indices=2  OutputSizes=1
  Terminator{,2..5} (5 alike) : Terminator
  To Workspace : ToWorkspace  VariableName=airspeed  SaveFormat=Timeseries  SampleTime=-1
  out : Outport
  wires:
  "6DOF Rigid body dynamics "/9 -> Bus Creator/8  "Vb_dot"
  Selector/1 -> ISA Atmosphere Model/1
  "6DOF Rigid body dynamics "/3 -> Force and Moment Calculation/5(rpy), Bus Creator/4  "phithetapsi"
  Constant/1 -> Flat Earth to LLA/2
  Constant2/1 -> Bus Creator/10  "B"
  "6DOF Rigid body dynamics "/5 -> Bus Creator/6  "Vb"
  ISA Atmosphere Model/3 -> Bus Creator/12  "P_inf"
  ISA Atmosphere Model/2 -> Bus Creator/16, Terminator4/1  "a_inf"
  Bus Creator/1 -> out/1
  ISA Atmosphere Model/1 -> Bus Creator/11  "T_inf"
  "6DOF Rigid body dynamics "/4 -> Bus Creator/5, Force and Moment Calculation/1(DCMbe)  "DCMbe"
  "6DOF Rigid body dynamics "/6 -> Force and Moment Calculation/4(pqr_b), Bus Creator/7  "omega_b"
  Force and Moment Calculation/1(F_xyz) -> "6DOF Rigid body dynamics "/1
  "6DOF Rigid body dynamics "/1 -> Bus Creator/2, Force and Moment Calculation/2(Ve)  "Vbned"
  Flat Earth to LLA/1 -> Mux/1
  Flat Earth to LLA/2 -> Mux/2
  Constant3/1 -> Bus Creator/14  "Vw"
  Force and Moment Calculation/2(M_xyz) -> "6DOF Rigid body dynamics "/2
  "6DOF Rigid body dynamics "/8 -> Terminator5/1
  [mulh] -> Selector/1
  "6DOF Rigid body dynamics "/7 -> Terminator3/1
  pwm/1 -> Force and Moment Calculation/6(Inputs)
  "6DOF Rigid body dynamics "/2 -> Flat Earth to LLA/1, Bus Creator/3, Force and Moment Calculation/3(Xe)  "xyzned"
  Force and Moment Calculation/3(Airspeed) -> Bus Creator/15, To Workspace/1  "airspeed"
  ISA Atmosphere Model/4 -> Bus Creator/13  "rho_inf"
  Mux/1 -> Bus Creator/1, [mulh]  "mulh"
  Constant1/1 -> Bus Creator/9  "g"
  ? -> Terminator/1
  ? -> Terminator2/1

== system FixedWing_Dynamic_Model_SIL_simulink/Dynamics/save to file ==
  pwm : Inport
  out : Inport  Port=2
  To File : ToFile  Filename=simulacionSimulink_out  SaveFormat=Timeseries
  To File1 : ToFile  Filename=simulacionSimulink_PWM  SaveFormat=Timeseries
  wires:
  out/1 -> To File/1
  pwm/1 -> To File1/1

== system FixedWing_Dynamic_Model_SIL_simulink/Controllers/Attitude Controller/Mix (control allocation) ==
  In1 : Inport  SampleTime=frecuency
  Constant : Constant  Value=[1,0,0;0,1,0;0,0,1]  SampleTime=frecuency
  MatrixMultiply : Product  Multiplication=Matrix(*)
  Out1 : Outport  SampleTime=frecuency
  wires:
  Constant/1 -> MatrixMultiply/1
  In1/1 -> MatrixMultiply/2
  MatrixMultiply/1 -> Out1/1

== system FixedWing_Dynamic_Model_SIL_simulink/Controllers/Attitude Controller/Scaler_1 ==
  ff : Inport  SampleTime=frecuency
  VTAS_sp : Inport  Port=2  SampleTime=frecuency
  V_TAS : Inport  Port=3  SampleTime=frecuency
  Product : Product  Inputs=**/
  Out1 : Outport  SampleTime=frecuency
  wires:
  VTAS_sp/1 -> Product/2
  ff/1 -> Product/1
  V_TAS/1 -> Product/3
  Product/1 -> Out1/1

== system FixedWing_Dynamic_Model_SIL_simulink/Controllers/Attitude Controller/Scaler_2 ==
  V_TAS : Inport  SampleTime=frecuency
  VTAS_sp : Inport  Port=2  SampleTime=frecuency
  PI : Inport  Port=3  SampleTime=frecuency
  Product : Product  Inputs=***//
  Out1 : Outport  SampleTime=frecuency
  wires:
  VTAS_sp/1 -> Product/3, Product/2
  PI/1 -> Product/1
  Product/1 -> Out1/1
  V_TAS/1 -> Product/5, Product/4

== system FixedWing_Dynamic_Model_SIL_simulink/Controllers/Attitude Controller/Subsystem ==
  In1 : Inport  SampleTime=frecuency
  Demux : Demux  Outputs=3
  Gain : Gain  Gain=roll_ff
  Gain1 : Gain  Gain=pitch_ff
  Gain2 : Gain  Gain=yaw_ff
  Mux : Mux  Inputs=3
  Out1 : Outport  SampleTime=frecuency
  wires:
  In1/1 -> Demux/1
  Demux/1 -> Gain/1
  Demux/2 -> Gain1/1
  Demux/3 -> Gain2/1
  Gain/1 -> Mux/1
  Gain1/1 -> Mux/2
  Gain2/1 -> Mux/3
  Mux/1 -> Out1/1

== system FixedWing_Dynamic_Model_SIL_simulink/Controllers/Attitude Controller/Subsystem1 ==
  In1 : Inport  SampleTime=frecuency
  Demux : Demux  Outputs=3
  Mux : Mux  Inputs=3
  PID Controller : slpidlib/PID Controller  Controller=PID  Form=Parallel  TimeDomain=Discrete-time  UseExternalTs=off  SampleTime=frecuency  IntegratorMethod=Forward Euler  FilterMethod=Forward Euler  ControllerParametersSource=internal  P=roll_P  I=roll_I  UseKiTs=off  D=roll_D  N=100  UseFilter=on  TunerSelectOption=Transfer Function Based (PID Tuner App)  InitialConditionSource=internal  InitialConditionForIntegrator=0  InitialConditionForFilter=0  DifferentiatorICPrevScaledInput=0  ExternalReset=none  TrackingMode=off  Kt=1  LimitOutput=off  SatLimitsSource=internal  UpperSaturationLimit=inf  LowerSaturationLimit=-inf  LinearizeAsGain=on  AntiWindupMode=none  Kb=1  LimitIntegrator=off  UpperIntegratorSaturationLimit=inf  LowerIntegratorSaturationLimit=-inf  POutMin=[]  POutMax=[]  IOutMin=[]  IOutMax=[]  DOutMin=[]  DOutMax=[]  NOutMin=[]  NOutMax=[]  SumOutMin=[]  SumOutMax=[]  SaturationOutMin=[]  SaturationOutMax=[]  PParamMin=[]  PParamMax=[]  IParamMin=[]  IParamMax=[]  DParamMin=[]  DParamMax=[]  NParamMin=[]  NParamMax=[]  KbParamMin=[]  KbParamMax=[]  KtParamMin=[]  KtParamMax=[]  KbOutMin=[]  KbOutMax=[]  KtOutMin=[]  KtOutMax=[]  IntegratorOutMin=[]  IntegratorOutMax=[]  FilterOutMin=[]  FilterOutMax=[]  SumI1OutMin=[]  SumI1OutMax=[]  SumI2OutMin=[]  SumI2OutMax=[]  SumI3OutMin=[]  SumI3OutMax=[]  SumI4OutMin=[]  SumI4OutMax=[]  SumDOutMin=[]  SumDOutMax=[]  DifferentiatorOutMin=[]  DifferentiatorOutMax=[]  FilterDiffOutCoefMin=[]  FilterDiffOutCoefMax=[]  ReciprocalOutMin=[]  ReciprocalOutMax=[]  SumDenOutMin=[]  SumDenOutMax=[]  SumNumOutMin=[]  SumNumOutMax=[]  DivideOutMin=[]  DivideOutMax=[]  UdiffTsProdOutMin=[]  UdiffTsProdOutMax=[]  NTsProdOutMin=[]  NTsProdOutMax=[]  UintegralTsProdOutMin=[]  UintegralTsProdOutMax=[]  UngainTsProdOutMin=[]  UngainTsProdOutMax=[]  ClampingZeroOutDataTypeStr=Inherit: Inherit via back propagation  ClampingZeroOutMin=[]  ClampingZeroOutMax=[]  FilterDenConstantOutDataTypeStr=Inherit: Inherit via back propagation  FilterDenConstantOutMin=[]  FilterDenConstantOutMax=[]  PCopyOutDataTypeStr=Inherit: Inherit via back propagation  PCopyOutMin=[]  PCopyOutMax=[]  NCopyOutDataTypeStr=Inherit: Inherit via back propagation  NCopyOutMin=[]  NCopyOutMax=[]  IntegratorContinuousStateAttributes=''  IntegratorStateMustResolveToSignalObject=off  IntegratorRTWStateStorageClass=Auto  FilterContinuousStateAttributes=''  FilterStateMustResolveToSignalObject=off  FilterRTWStateStorageClass=Auto  ParallelPVariant=InternalParameters  IdealPVariant=Disabled  IVariant=InternalParameters  DVariant=InternalParameters  IntegratorVariant=Discrete  SatVariant=Disabled  AWVariant=Passthrough  PCopyVariant=Disabled  TRVariant=Disabled  FdbkBlocksVariant=Forward  IdealPFdbkVariant=Disabled  SatFdbkVariant=Disabled  DerivativeFilterVariant=ForwardEulerFilter  NVariant=InternalParameters  NCopyVariant=Disabled  FilterICVariant=InternalICsFilter  IntegratorICVariant=InternalICs  ExternalResetVariant=Disabled  TRSumVariant=Passthrough  SumFdbkVariant=Disabled  SumVariant=Sum_PID  TsampFilterVariant=InternalTs  TsampNgainVariant=Passthrough  TsampIntegralVariant=Disabled_SignalSpec  ExternalSaturationOutDataTypeStr=Inherit: Same as second input
  PID Controller1 : slpidlib/PID Controller  Controller=PID  Form=Parallel  TimeDomain=Discrete-time  UseExternalTs=off  SampleTime=frecuency  IntegratorMethod=Forward Euler  FilterMethod=Forward Euler  ControllerParametersSource=internal  P=pitch_P  I=pitch_I  UseKiTs=off  D=pitch_D  N=100  UseFilter=on  TunerSelectOption=Transfer Function Based (PID Tuner App)  InitialConditionSource=internal  InitialConditionForIntegrator=0  InitialConditionForFilter=0  DifferentiatorICPrevScaledInput=0  ExternalReset=none  TrackingMode=off  Kt=1  LimitOutput=off  SatLimitsSource=internal  UpperSaturationLimit=inf  LowerSaturationLimit=-inf  LinearizeAsGain=on  AntiWindupMode=none  Kb=1  LimitIntegrator=off  UpperIntegratorSaturationLimit=inf  LowerIntegratorSaturationLimit=-inf  POutMin=[]  POutMax=[]  IOutMin=[]  IOutMax=[]  DOutMin=[]  DOutMax=[]  NOutMin=[]  NOutMax=[]  SumOutMin=[]  SumOutMax=[]  SaturationOutMin=[]  SaturationOutMax=[]  PParamMin=[]  PParamMax=[]  IParamMin=[]  IParamMax=[]  DParamMin=[]  DParamMax=[]  NParamMin=[]  NParamMax=[]  KbParamMin=[]  KbParamMax=[]  KtParamMin=[]  KtParamMax=[]  KbOutMin=[]  KbOutMax=[]  KtOutMin=[]  KtOutMax=[]  IntegratorOutMin=[]  IntegratorOutMax=[]  FilterOutMin=[]  FilterOutMax=[]  SumI1OutMin=[]  SumI1OutMax=[]  SumI2OutMin=[]  SumI2OutMax=[]  SumI3OutMin=[]  SumI3OutMax=[]  SumI4OutMin=[]  SumI4OutMax=[]  SumDOutMin=[]  SumDOutMax=[]  DifferentiatorOutMin=[]  DifferentiatorOutMax=[]  FilterDiffOutCoefMin=[]  FilterDiffOutCoefMax=[]  ReciprocalOutMin=[]  ReciprocalOutMax=[]  SumDenOutMin=[]  SumDenOutMax=[]  SumNumOutMin=[]  SumNumOutMax=[]  DivideOutMin=[]  DivideOutMax=[]  UdiffTsProdOutMin=[]  UdiffTsProdOutMax=[]  NTsProdOutMin=[]  NTsProdOutMax=[]  UintegralTsProdOutMin=[]  UintegralTsProdOutMax=[]  UngainTsProdOutMin=[]  UngainTsProdOutMax=[]  ClampingZeroOutDataTypeStr=Inherit: Inherit via back propagation  ClampingZeroOutMin=[]  ClampingZeroOutMax=[]  FilterDenConstantOutDataTypeStr=Inherit: Inherit via back propagation  FilterDenConstantOutMin=[]  FilterDenConstantOutMax=[]  PCopyOutDataTypeStr=Inherit: Inherit via back propagation  PCopyOutMin=[]  PCopyOutMax=[]  NCopyOutDataTypeStr=Inherit: Inherit via back propagation  NCopyOutMin=[]  NCopyOutMax=[]  IntegratorContinuousStateAttributes=''  IntegratorStateMustResolveToSignalObject=off  IntegratorRTWStateStorageClass=Auto  FilterContinuousStateAttributes=''  FilterStateMustResolveToSignalObject=off  FilterRTWStateStorageClass=Auto  ParallelPVariant=InternalParameters  IdealPVariant=Disabled  IVariant=InternalParameters  DVariant=InternalParameters  IntegratorVariant=Discrete  SatVariant=Disabled  AWVariant=Passthrough  PCopyVariant=Disabled  TRVariant=Disabled  FdbkBlocksVariant=Forward  IdealPFdbkVariant=Disabled  SatFdbkVariant=Disabled  DerivativeFilterVariant=ForwardEulerFilter  NVariant=InternalParameters  NCopyVariant=Disabled  FilterICVariant=InternalICsFilter  IntegratorICVariant=InternalICs  ExternalResetVariant=Disabled  TRSumVariant=Passthrough  SumFdbkVariant=Disabled  SumVariant=Sum_PID  TsampFilterVariant=InternalTs  TsampNgainVariant=Passthrough  TsampIntegralVariant=Disabled_SignalSpec  ExternalSaturationOutDataTypeStr=Inherit: Same as second input
  PID Controller2 : slpidlib/PID Controller  Controller=PID  Form=Parallel  TimeDomain=Discrete-time  UseExternalTs=off  SampleTime=frecuency  IntegratorMethod=Forward Euler  FilterMethod=Forward Euler  ControllerParametersSource=internal  P=yaw_P  I=yaw_I  UseKiTs=off  D=yaw_D  N=100  UseFilter=on  TunerSelectOption=Transfer Function Based (PID Tuner App)  InitialConditionSource=internal  InitialConditionForIntegrator=0  InitialConditionForFilter=0  DifferentiatorICPrevScaledInput=0  ExternalReset=none  TrackingMode=off  Kt=1  LimitOutput=off  SatLimitsSource=internal  UpperSaturationLimit=inf  LowerSaturationLimit=-inf  LinearizeAsGain=on  AntiWindupMode=none  Kb=1  LimitIntegrator=off  UpperIntegratorSaturationLimit=inf  LowerIntegratorSaturationLimit=-inf  POutMin=[]  POutMax=[]  IOutMin=[]  IOutMax=[]  DOutMin=[]  DOutMax=[]  NOutMin=[]  NOutMax=[]  SumOutMin=[]  SumOutMax=[]  SaturationOutMin=[]  SaturationOutMax=[]  PParamMin=[]  PParamMax=[]  IParamMin=[]  IParamMax=[]  DParamMin=[]  DParamMax=[]  NParamMin=[]  NParamMax=[]  KbParamMin=[]  KbParamMax=[]  KtParamMin=[]  KtParamMax=[]  KbOutMin=[]  KbOutMax=[]  KtOutMin=[]  KtOutMax=[]  IntegratorOutMin=[]  IntegratorOutMax=[]  FilterOutMin=[]  FilterOutMax=[]  SumI1OutMin=[]  SumI1OutMax=[]  SumI2OutMin=[]  SumI2OutMax=[]  SumI3OutMin=[]  SumI3OutMax=[]  SumI4OutMin=[]  SumI4OutMax=[]  SumDOutMin=[]  SumDOutMax=[]  DifferentiatorOutMin=[]  DifferentiatorOutMax=[]  FilterDiffOutCoefMin=[]  FilterDiffOutCoefMax=[]  ReciprocalOutMin=[]  ReciprocalOutMax=[]  SumDenOutMin=[]  SumDenOutMax=[]  SumNumOutMin=[]  SumNumOutMax=[]  DivideOutMin=[]  DivideOutMax=[]  UdiffTsProdOutMin=[]  UdiffTsProdOutMax=[]  NTsProdOutMin=[]  NTsProdOutMax=[]  UintegralTsProdOutMin=[]  UintegralTsProdOutMax=[]  UngainTsProdOutMin=[]  UngainTsProdOutMax=[]  ClampingZeroOutDataTypeStr=Inherit: Inherit via back propagation  ClampingZeroOutMin=[]  ClampingZeroOutMax=[]  FilterDenConstantOutDataTypeStr=Inherit: Inherit via back propagation  FilterDenConstantOutMin=[]  FilterDenConstantOutMax=[]  PCopyOutDataTypeStr=Inherit: Inherit via back propagation  PCopyOutMin=[]  PCopyOutMax=[]  NCopyOutDataTypeStr=Inherit: Inherit via back propagation  NCopyOutMin=[]  NCopyOutMax=[]  IntegratorContinuousStateAttributes=''  IntegratorStateMustResolveToSignalObject=off  IntegratorRTWStateStorageClass=Auto  FilterContinuousStateAttributes=''  FilterStateMustResolveToSignalObject=off  FilterRTWStateStorageClass=Auto  ParallelPVariant=InternalParameters  IdealPVariant=Disabled  IVariant=InternalParameters  DVariant=InternalParameters  IntegratorVariant=Discrete  SatVariant=Disabled  AWVariant=Passthrough  PCopyVariant=Disabled  TRVariant=Disabled  FdbkBlocksVariant=Forward  IdealPFdbkVariant=Disabled  SatFdbkVariant=Disabled  DerivativeFilterVariant=ForwardEulerFilter  NVariant=InternalParameters  NCopyVariant=Disabled  FilterICVariant=InternalICsFilter  IntegratorICVariant=InternalICs  ExternalResetVariant=Disabled  TRSumVariant=Passthrough  SumFdbkVariant=Disabled  SumVariant=Sum_PID  TsampFilterVariant=InternalTs  TsampNgainVariant=Passthrough  TsampIntegralVariant=Disabled_SignalSpec  ExternalSaturationOutDataTypeStr=Inherit: Same as second input
  Out1 : Outport  SampleTime=frecuency
  wires:
  Demux/1 -> PID Controller/1
  PID Controller1/1 -> Mux/2
  Mux/1 -> Out1/1
  PID Controller/1 -> Mux/1
  In1/1 -> Demux/1
  Demux/2 -> PID Controller1/1
  PID Controller2/1 -> Mux/3
  Demux/3 -> PID Controller2/1

== system FixedWing_Dynamic_Model_SIL_simulink/Controllers/Attitude Controller/Subsystem2 ==
  In1 : Inport
  Demux : Demux  Outputs=3
  Mux : Mux  Inputs=3
  Saturation1 : Saturate  UpperLimit=1  LowerLimit=-1
  Saturation2 : Saturate  UpperLimit=1  LowerLimit=-1
  Saturation3 : Saturate  UpperLimit=1  LowerLimit=-1
  Out1 : Outport
  wires:
  In1/1 -> Demux/1
  Mux/1 -> Out1/1
  Demux/1 -> Saturation3/1
  Saturation1/1 -> Mux/3
  Demux/3 -> Saturation1/1
  Saturation2/1 -> Mux/1
  Saturation3/1 -> Mux/2
  Demux/2 -> Saturation2/1

== system FixedWing_Dynamic_Model_SIL_simulink/Controllers/Attitude Controller/Subsystem3 ==
  In1 : Inport  SampleTime=frecuency
  In2 : Inport  Port=2  SampleTime=frecuency
  Add : Sum  Inputs=+-
  Add1 : Sum  Inputs=+-
  Add2 : Sum  Inputs=+-
  Demux : Demux  Outputs=3
  Demux1 : Demux  Outputs=3
  Mux : Mux  Inputs=3
  Out1 : Outport  SampleTime=frecuency
  wires:
  Demux/1 -> Add/1
  Demux/2 -> Add1/1
  Demux/3 -> Add2/1
  Demux1/1 -> Add/2
  Demux1/2 -> Add1/2
  Demux1/3 -> Add2/2
  In1/1 -> Demux/1
  Add/1 -> Mux/1
  Add1/1 -> Mux/2
  Add2/1 -> Mux/3
  Mux/1 -> Out1/1
  In2/1 -> Demux1/1

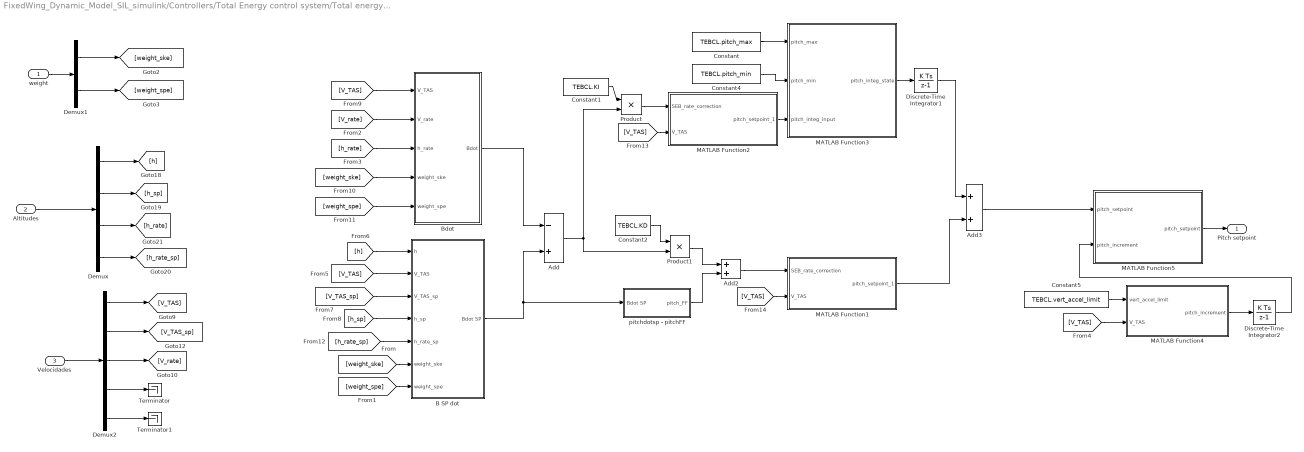
== system FixedWing_Dynamic_Model_SIL_simulink/Controllers/Total Energy control system/Total energy balance control loop ==
  weight : Inport  SampleTime=frecuency
  Altitudes : Inport  Port=2  SampleTime=frecuency
  Velocidades : Inport  Port=3  SampleTime=frecuency
  " B SP dot" : Subsystem
  Add : Sum  Inputs=-+
  Add2 : Sum
  Add3 : Sum
  Bdot : Subsystem
  Constant : Constant  Value=TEBCL.pitch_max  SampleTime=frecuency
  Constant1 : Constant  Value=TEBCL.KI  SampleTime=frecuency
  Constant2 : Constant  Value=TEBCL.KD  SampleTime=frecuency
  Constant4 : Constant  Value=TEBCL.pitch_min  SampleTime=frecuency
  Constant5 : Constant  Value=TEBCL.vert_accel_limit  SampleTime=frecuency
  Demux : Demux
  Demux1 : Demux  Outputs=2
  Demux2 : Demux  Outputs=5
  Discrete-Time Integrator1 : DiscreteIntegrator  SampleTime=frecuency  ICPrevOutput=DiscIntNeverNeededParam  ICPrevScaledInput=DiscIntNeverNeededParam
  Discrete-Time Integrator2 : DiscreteIntegrator  SampleTime=frecuency  ICPrevOutput=DiscIntNeverNeededParam  ICPrevScaledInput=DiscIntNeverNeededParam
  MATLAB Function1 : MATLAB Function  TreatAsAtomicUnit=on  SystemSampleTime=frecuency
  MATLAB Function2 : MATLAB Function  TreatAsAtomicUnit=on  SystemSampleTime=frecuency
  MATLAB Function3 : MATLAB Function  TreatAsAtomicUnit=on  SystemSampleTime=frecuency
  MATLAB Function4 : MATLAB Function  TreatAsAtomicUnit=on  SystemSampleTime=frecuency
  MATLAB Function5 : MATLAB Function  TreatAsAtomicUnit=on  SystemSampleTime=frecuency
  Product : Product
  Product1 : Product
  Terminator : Terminator
  Terminator1 : Terminator
  pitchdotsp - pitchFF : Subsystem
  Pitch setpoint : Outport  SampleTime=frecuency
  wires:
  Add/1 -> Product1/2, Product/2
  [V_TAS] -> Bdot/1(V_TAS)
  [h_sp] -> " B SP dot"/4(h_sp)
  [V_TAS_sp] -> " B SP dot"/3(V_TAS_sp)
  [h] -> " B SP dot"/1(h)
  [V_TAS] -> " B SP dot"/2(V_TAS)
  Bdot/1(Bdot) -> Add/1
  " B SP dot"/1(Bdot SP) -> Add/2, pitchdotsp - pitchFF/1(Bdot SP)
  [weight_ske] -> " B SP dot"/6(weight_ske)
  [weight_spe] -> " B SP dot"/7(weight_spe)
  [weight_spe] -> Bdot/5(weight_spe)
  [weight_ske] -> Bdot/4(weight_ske)
  [h_rate] -> Bdot/3(h_rate)
  [V_rate] -> Bdot/2(V_rate)
  [h_rate_sp] -> " B SP dot"/5(h_rate_sp)
  Add3/1 -> MATLAB Function5/1("pitch_setpoint ")
  MATLAB Function1/1(pitch_setpoint_1) -> Add3/2
  Product/1 -> MATLAB Function2/1(SEB_rate_correction)
  [V_TAS] -> MATLAB Function2/2(V_TAS)
  Product1/1 -> Add2/1
  pitchdotsp - pitchFF/1(pitch_FF) -> Add2/2
  Add2/1 -> MATLAB Function1/1(SEB_rate_correction)
  [V_TAS] -> MATLAB Function1/2(V_TAS)
  Constant1/1 -> Product/1
  Constant2/1 -> Product1/1
  MATLAB Function3/1(pitch_integ_state) -> Discrete-Time Integrator1/1
  MATLAB Function2/1(pitch_setpoint_1) -> MATLAB Function3/3(pitch_integ_input)
  Constant4/1 -> MATLAB Function3/2(pitch_min)
  Constant/1 -> MATLAB Function3/1(pitch_max)
  Constant5/1 -> MATLAB Function4/1(vert_accel_limit)
  [V_TAS] -> MATLAB Function4/2(V_TAS)
  MATLAB Function4/1(pitch_increment) -> Discrete-Time Integrator2/1
  MATLAB Function5/1(pitch_setpoint) -> Pitch setpoint/1
  Discrete-Time Integrator2/1 -> MATLAB Function5/2(pitch_increment)
  Demux2/5 -> Terminator1/1
  Velocidades/1 -> Demux2/1
  Demux/4 -> [h_rate_sp]
  Demux2/4 -> Terminator/1
  Demux2/1 -> [V_TAS]
  Demux/1 -> [h]
  Demux2/2 -> [V_TAS_sp]
  Demux2/3 -> [V_rate]
  Demux/3 -> [h_rate]
  Altitudes/1 -> Demux/1
  Demux/2 -> [h_sp]
  Demux1/1 -> [weight_ske]
  weight/1 -> Demux1/1
  Demux1/2 -> [weight_spe]
  Discrete-Time Integrator1/1 -> Add3/1
